simulink model "lab4_1_3"  (R2022a)
settings: Solver=VariableStepAuto  StartTime=0.0  StopTime=Tmdl  FixedStep=To/100  MaxStep=To/100  RelTol=1e-3
undefined symbols (not defined in the file or in its folder): an, dsc, T, To
settings Model: Creator=Professional  LastModifiedBy=osini

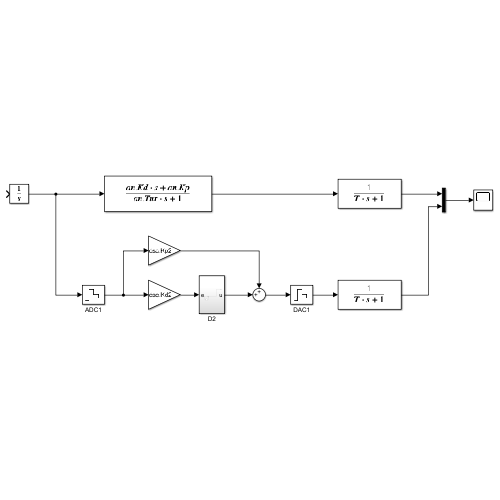
[thumbnail: Simulink's stored preview of the top-level diagram]
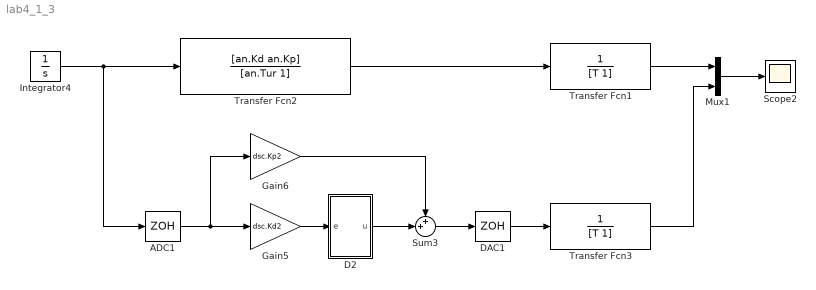
== system lab4_1_3 ==
  ADC1 : ZeroOrderHold  SampleTime=To
  D2 : Subsystem
  DAC1 : ZeroOrderHold  SampleTime=To
  Gain5 : Gain  Gain=dsc.Kd2
  Gain6 : Gain  Gain=dsc.Kp2
  Integrator4 : Integrator  InitialCondition=1
  Mux1 : Mux  Inputs=2
  Scope2 : Scope
  Sum3 : Sum  Inputs=++|
  Transfer Fcn1 : TransferFcn  Denominator=[T 1]
  Transfer Fcn2 : TransferFcn  Numerator=[an.Kd an.Kp]  Denominator=[an.Tur 1]
  Transfer Fcn3 : TransferFcn  Denominator=[T 1]
  wires:
  Mux1/1 -> Scope2/1
  Transfer Fcn1/1 -> Mux1/1
  ADC1/1 -> Gain6/1, Gain5/1
  Transfer Fcn3/1 -> Mux1/2
  Gain5/1 -> D2/1(e)
  Integrator4/1 -> Transfer Fcn2/1, ADC1/1
  DAC1/1 -> Transfer Fcn3/1
  Gain6/1 -> Sum3/1
  D2/1(u) -> Sum3/2
  Sum3/1 -> DAC1/1
  Transfer Fcn2/1 -> Transfer Fcn1/1

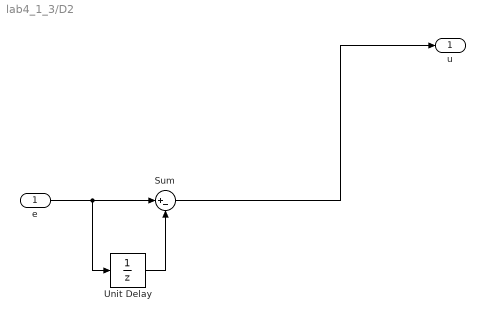
== system lab4_1_3/D2 ==
  e : Inport
  Sum : Sum  Inputs=|+-
  Unit Delay : UnitDelay  SampleTime=-1  HasFrameUpgradeWarning=on
  u : Outport
  wires:
  e/1 -> Unit Delay/1, Sum/1
  Unit Delay/1 -> Sum/2
  Sum/1 -> u/1
